simulink model "FG_Simulator"  (R2017b)
settings: Solver=ode45  StartTime=0  StopTime=20  FixedStep=0.0005  EnableMultiTasking=on
InitFcn:
  | isSim = 1;
  | 
  | PreFunctions.CustomInitFcn;
  | PreFunctions.simulationInitFcn
undefined symbols (not defined in the file): DiagnosticCodes, motorPositions, motorVelocities, pelvisPosition, pelvisVelocity, sample_time, X, Y, Z
libraries: sm_lib x170, nesl_utility x75, Contact_Forces_Lib x6, ComponentLibrary x5, Cassie_CommandBlock_Library_3 x1, Cassie_CommandBlock_Library_5 x1
(part 1 of 7)
settings Model: Creator=case  LastModifiedBy=81068
settings SolverCC: ZeroCrossControl=DisableAll  InsertRTBMode=Always
settings DataIOCC: SaveOutput=off  SignalLogging=off  DSMLogging=off  SaveTime=off
settings OptimizationCC: DefaultParameterBehavior=Inlined  UseFloatMulNetSlope=on  InlineInvariantSignals=on  EfficientFloat2IntCast=on  LifeSpan=inf  SimCompilerOptimization=on  AccelVerboseBuild=on
settings DebuggingCC: ReadBeforeWriteMsg=DisableAll  WriteAfterWriteMsg=DisableAll  WriteAfterReadMsg=DisableAll  ParameterUnderflowMsg=error  ParameterTunabilityLossMsg=error  UniqueDataStoreMsg=error  AllowSymbolicDim=off  StrictBusMsg=ErrorOnBusTreatedAsVector  SFUnexpectedBacktrackingDiag=warning  SFNoUnconditionalDefaultTransitionDiag=warning  SFExecutionAtInitializationDiag=none
settings HardwareCC: TargetBitPerPointer=64  TargetBitPerSizeT=64  TargetBitPerPtrDiffT=64  TargetLongLongMode=on  TargetIntDivRoundTo=Zero  TargetEndianess=LittleEndian  TargetWordSize=64  TargetHWDeviceType=MATLAB Host  ProdEqTarget=off
settings ModelReferenceCC: EnableParallelModelReferenceBuilds=on  ModelReferenceNumInstancesAllowed=Zero  ModelReferenceMinAlgLoopOccurrences=on  PropagateSignalLabelsOutOfModel=off
settings SFSimCC: SimUserIncludeDirs=$root_dir$\CustomCodes\utils\funcs\KinDyn200511_221619
settings SFSimCC: SimUserSources=|
  | R_LeftAbductionJoint_src.c
  | R_LeftThighJoint_src.c
  | R_RightAbductionJoint_src.c
  | R_RightThighJoint_src.c
  | 
  | AMworld_about_pA_src.c
  | 
  | Jb_BasePosX_src.c
  | Jb_BasePosY_src.c
  | Jb_BasePosZ_src.c
  | Jb_BaseRotX_src.c
  | Jb_BaseRotY_src.c
  | Jb_BaseRotZ_src.c
  | Jb_LeftAbductionJoint_src.c
  | Jb_LeftAnkleJoint_src.c
  | Jb_LeftHip_src.c
  | Jb_LeftKneeJoint_src.c
  | Jb_LeftKneeSpringJoint_src.c
  | Jb_LeftKnee_src.c
  | Jb_LeftPelvisRotation_src.c
  | Jb_LeftRotationJoint_src.c
  | Jb_LeftShin_src.c
  | Jb_LeftTarsus_src.c
  | Jb_LeftThighJoint_src.c
  | Jb_LeftThigh_src.c
  | Jb_LeftToeBottomBack_src.c
  | Jb_LeftToeBottomFront_src.c
  | Jb_LeftToeBottom_src.c
  | Jb_LeftToeJoint_src.c
  | Jb_LeftToe_src.c
  | Jb_Pelvis_src.c
  | Jb_RightAbductionJoint_src.c
  | Jb_RightAnkleJoint_src.c
  | Jb_RightHip_src.c
  | Jb_RightKneeJoint_src.c
  | Jb_RightKneeSpringJoint_src.c
  | Jb_RightKnee_src.c
  | Jb_RightPelvisRotation_src.c
  | Jb_RightRotationJoint_src.c
  | Jb_RightShin_src.c
  | Jb_RightTarsus_src.c
  | Jb_RightThighJoint_src.c
  | Jb_RightThigh_src.c
  | Jb_RightToeBottomBack_src.c
  | Jb_RightToeBottomFront_src.c
  | Jb_RightToeBottom_src.c
  | Jb_RightToeJoint_src.c
  | Jb_RightToe_src.c
  | 
  | Jdq_AMworld_about_pA_src.c
  | 
  | 
  | Jp_COM_src.c
  | Jp_LeftAbductionJoint_src.c
  | Jp_LeftAnkleJoint_src.c
  | Jp_LeftHip_src.c
  | Jp_LeftKneeJoint_src.c
  | Jp_LeftKneeSpringJoint_src.c
  | Jp_LeftKnee_src.c
  | Jp_LeftPelvisRotation_src.c
  | Jp_LeftRotationJoint_src.c
  | Jp_LeftShin_src.c
  | Jp_LeftTarsus_src.c
  | Jp_LeftThighJoint_src.c
  | Jp_LeftThigh_src.c
  | Jp_LeftToeBottomBack_src.c
  | Jp_LeftToeBottomFront_src.c
  | Jp_LeftToeBottom_src.c
  | Jp_LeftToeJoint_src.c
  | Jp_LeftToe_src.c
  | Jp_Pelvis_src.c
  | Jp_RightAbductionJoint_src.c
  | Jp_RightAnkleJoint_src.c
  | Jp_RightHip_src.c
  | Jp_RightKneeJoint_src.c
  | Jp_RightKneeSpringJoint_src.c
  | Jp_RightKnee_src.c
  | Jp_RightPelvisRotation_src.c
  | Jp_RightRotationJoint_src.c
  | Jp_RightShin_src.c
  | Jp_RightTarsus_src.c
  | Jp_RightThighJoint_src.c
  | Jp_RightThigh_src.c
  | Jp_RightToeBottomBack_src.c
  | Jp_RightToeBottomFront_src.c
  | Jp_RightToeBottom_src.c
  | Jp_RightToeJoint_src.c
  | Jp_RightToe_src.c
  | 
  | p_BasePosX_src.c
  | p_BasePosY_src.c
  | p_BasePosZ_src.c
  | p_BaseRotX_src.c
  | p_BaseRotY_src.c
  | p_BaseRotZ_src.c
  | p_COM_src.c
  | p_LeftAbductionJoint_src.c
  | p_LeftAnkleJoint_src.c
  | p_LeftHip_src.c
  | p_LeftKneeJoint_src.c
  | p_LeftKneeSpringJoint_src.c
  | p_LeftKnee_src.c
  | p_LeftPelvisRotation_src.c
  | p_LeftRotationJoint_src.c
  | p_LeftShin_src.c
  | p_LeftTarsus_src.c
  | p_LeftThighJoint_src.c
  | p_LeftThigh_src.c
  | p_LeftToeBottomBack_src.c
  | p_LeftToeBottomFront_src.c
  | p_LeftToeBottom_src.c
  | p_LeftToeJoint_src.c
  | p_LeftToe_src.c
  | p_Pelvis_src.c
  | p_RightAbductionJoint_src.c
  | p_RightAnkleJoint_src.c
  | p_RightHip_src.c
  | p_RightKneeJoint_src.c
  | p_RightKneeSpringJoint_src.c
  | p_RightKnee_src.c
  | p_RightPelvisRotation_src.c
  | p_RightRotationJoint_src.c
  | p_RightShin_src.c
  | p_RightTarsus_src.c
  | p_RightThighJoint_src.c
  | p_RightThigh_src.c
  | p_RightToeBottomBack_src.c
  | p_RightToeBottomFront_src.c
  | p_RightToeBottom_src.c
  | p_RightToeJoint_src.c
  | p_RightToe_src.c
  | 
  | T_LeftToeBottomBack_src.c
  | T_LeftToeBottomFront_src.c
  | T_LeftToeBottom_src.c
  | T_RightToeBottomBack_src.c
  | T_RightToeBottomFront_src.c
  | T_RightToeBottom_src.c
  | 
  | J_LL_Left_src.c
  | J_LL_Right_src.c
  | LL_Left_src.c
  | LL_Right_src.c
settings RTWCC: Description=Generic Real-Time Target  RTWUseSimCustomCode=on  CustomInclude=$root_dir$\CustomCodes\utils\funcs\KinDyn200511_221619  BuildConfiguration=Faster Runs  CheckMdlBeforeBuild=Warning
settings RTWCC: CustomSource=|
  | R_LeftAbductionJoint_src.c
  | R_LeftThighJoint_src.c
  | R_RightAbductionJoint_src.c
  | R_RightThighJoint_src.c
  | 
  | AMworld_about_pA_src.c
  | 
  | Jb_BasePosX_src.c
  | Jb_BasePosY_src.c
  | Jb_BasePosZ_src.c
  | Jb_BaseRotX_src.c
  | Jb_BaseRotY_src.c
  | Jb_BaseRotZ_src.c
  | Jb_LeftAbductionJoint_src.c
  | Jb_LeftAnkleJoint_src.c
  | Jb_LeftHip_src.c
  | Jb_LeftKneeJoint_src.c
  | Jb_LeftKneeSpringJoint_src.c
  | Jb_LeftKnee_src.c
  | Jb_LeftPelvisRotation_src.c
  | Jb_LeftRotationJoint_src.c
  | Jb_LeftShin_src.c
  | Jb_LeftTarsus_src.c
  | Jb_LeftThighJoint_src.c
  | Jb_LeftThigh_src.c
  | Jb_LeftToeBottomBack_src.c
  | Jb_LeftToeBottomFront_src.c
  | Jb_LeftToeBottom_src.c
  | Jb_LeftToeJoint_src.c
  | Jb_LeftToe_src.c
  | Jb_Pelvis_src.c
  | Jb_RightAbductionJoint_src.c
  | Jb_RightAnkleJoint_src.c
  | Jb_RightHip_src.c
  | Jb_RightKneeJoint_src.c
  | Jb_RightKneeSpringJoint_src.c
  | Jb_RightKnee_src.c
  | Jb_RightPelvisRotation_src.c
  | Jb_RightRotationJoint_src.c
  | Jb_RightShin_src.c
  | Jb_RightTarsus_src.c
  | Jb_RightThighJoint_src.c
  | Jb_RightThigh_src.c
  | Jb_RightToeBottomBack_src.c
  | Jb_RightToeBottomFront_src.c
  | Jb_RightToeBottom_src.c
  | Jb_RightToeJoint_src.c
  | Jb_RightToe_src.c
  | 
  | Jdq_AMworld_about_pA_src.c
  | 
  | 
  | Jp_COM_src.c
  | Jp_LeftAbductionJoint_src.c
  | Jp_LeftAnkleJoint_src.c
  | Jp_LeftHip_src.c
  | Jp_LeftKneeJoint_src.c
  | Jp_LeftKneeSpringJoint_src.c
  | Jp_LeftKnee_src.c
  | Jp_LeftPelvisRotation_src.c
  | Jp_LeftRotationJoint_src.c
  | Jp_LeftShin_src.c
  | Jp_LeftTarsus_src.c
  | Jp_LeftThighJoint_src.c
  | Jp_LeftThigh_src.c
  | Jp_LeftToeBottomBack_src.c
  | Jp_LeftToeBottomFront_src.c
  | Jp_LeftToeBottom_src.c
  | Jp_LeftToeJoint_src.c
  | Jp_LeftToe_src.c
  | Jp_Pelvis_src.c
  | Jp_RightAbductionJoint_src.c
  | Jp_RightAnkleJoint_src.c
  | Jp_RightHip_src.c
  | Jp_RightKneeJoint_src.c
  | Jp_RightKneeSpringJoint_src.c
  | Jp_RightKnee_src.c
  | Jp_RightPelvisRotation_src.c
  | Jp_RightRotationJoint_src.c
  | Jp_RightShin_src.c
  | Jp_RightTarsus_src.c
  | Jp_RightThighJoint_src.c
  | Jp_RightThigh_src.c
  | Jp_RightToeBottomBack_src.c
  | Jp_RightToeBottomFront_src.c
  | Jp_RightToeBottom_src.c
  | Jp_RightToeJoint_src.c
  | Jp_RightToe_src.c
  | 
  | p_BasePosX_src.c
  | p_BasePosY_src.c
  | p_BasePosZ_src.c
  | p_BaseRotX_src.c
  | p_BaseRotY_src.c
  | p_BaseRotZ_src.c
  | p_COM_src.c
  | p_LeftAbductionJoint_src.c
  | p_LeftAnkleJoint_src.c
  | p_LeftHip_src.c
  | p_LeftKneeJoint_src.c
  | p_LeftKneeSpringJoint_src.c
  | p_LeftKnee_src.c
  | p_LeftPelvisRotation_src.c
  | p_LeftRotationJoint_src.c
  | p_LeftShin_src.c
  | p_LeftTarsus_src.c
  | p_LeftThighJoint_src.c
  | p_LeftThigh_src.c
  | p_LeftToeBottomBack_src.c
  | p_LeftToeBottomFront_src.c
  | p_LeftToeBottom_src.c
  | p_LeftToeJoint_src.c
  | p_LeftToe_src.c
  | p_Pelvis_src.c
  | p_RightAbductionJoint_src.c
  | p_RightAnkleJoint_src.c
  | p_RightHip_src.c
  | p_RightKneeJoint_src.c
  | p_RightKneeSpringJoint_src.c
  | p_RightKnee_src.c
  | p_RightPelvisRotation_src.c
  | p_RightRotationJoint_src.c
  | p_RightShin_src.c
  | p_RightTarsus_src.c
  | p_RightThighJoint_src.c
  | p_RightThigh_src.c
  | p_RightToeBottomBack_src.c
  | p_RightToeBottomFront_src.c
  | p_RightToeBottom_src.c
  | p_RightToeJoint_src.c
  | p_RightToe_src.c
  | 
  | T_LeftToeBottomBack_src.c
  | T_LeftToeBottomFront_src.c
  | T_LeftToeBottom_src.c
  | T_RightToeBottomBack_src.c
  | T_RightToeBottomFront_src.c
  | T_RightToeBottom_src.c
  | 
  | J_LL_Left_src.c
  | J_LL_Right_src.c
  | LL_Left_src.c
  | LL_Right_src.c
settings CodeAppCC: GenerateComments=off  SimulinkBlockComments=off
settings GRTTargetCC: MatFileLogging=off  MultiInstanceERTCode=on  CodeInterfacePackaging=Reusable function  SupportNonFinite=off  GenerateAllocFcn=on
settings ConfigComp: CovMetricSettings=dw  CovHtmlReporting=on  CovSaveCumulativeToWorkspaceVar=on  CovSaveSingleToWorkspaceVar=on  CovExternalEMLEnable=off
settings SimscapeCC: SimscapeNormalizeSystem=off
settings DiagnosticsConfigSet: SimMechanicsRigidlyBoundBlock=warning
settings ExplorerConfigSet: InternalSimMechanicsExplorerSettings="<ExplorerConfiguration><canonicalview>default</canonicalview><AnimationSetting><BasePlaybackSpeed>1.0</BasePlaybackSpeed><PlaybackSpeedFactor>1.0</PlaybackSpeedFactor></AnimationSetting><TilePanel><TileInfo><Tiles Columns=\"1\" Count=\"1\" Rows=\"1\"><Column Weight=\"1\"/><Row Weight=\"1\"/><Tile Height=\"1\" Width=\"1\" X=\"0\" Y=\"0\"/></Tiles></TileInfo><SceneInfo><SceneViewer><BGColor><R>0.60000002384185791</R><G>0.60000002384185791</G><B>0.60000002384185791</B></BGColor><Camera><DoPerspective>off</DoPerspective><Position><X>-35.4589435173178984</X><Y>-0.0500115168093022214</Y><Z>0.273628552513051182</Z></Position><Center><X>1.71805707793737383e-06</X><Y>-0.0500115168093022214</Y><Z>0.273628552513051182</Z></Center><Up><X>0</X><Y>0</Y><Z>1</Z></Up><ViewLimDist>1</ViewLimDist><YLim>8.2670531882207996</YLim><XLim>14.7535103051325045</XLim></Camera></SceneViewer></SceneInfo></TilePanel><MechEditorPanel><Cameras><Camera><Id>Camera1</Id><Value><Name>Tracking Camera</Name><NativeCamera><PositionTrackingFeature>Cassie.Cassie_Simulation.World.Tracking_Camera.F</PositionTrackingFeature><CenterTrackingFeature>Cassie.Cassie_Simulation.World.Tracking_Camera_Target.F</CenterTrackingFeature><UpVectorTrackingFeature>Cassie.Cassie_Simulation.World.Tracking_Camera_Target.F</UpVectorTrackingFeature><CenterTrackingOrigin>on</CenterTrackingOrigin><UpVectorTrackingDirection>+Z</UpVectorTrackingDirection></NativeCamera></Value></Camera><Camera><Id>Camera2</Id><Value><Name>Fixed Camera</Name><NativeCamera><PositionTrackingFeature>Cassie.Cassie_Simulation.World.Fixed_Camera.F</PositionTrackingFeature><CenterTrackingFeature>Cassie.Cassie_Simulation.World.Fixed_Camera_Target.F</CenterTrackingFeature><UpVectorTrackingFeature>Cassie.Cassie_Simulation.World.Fixed_Camera_Target.F</UpVectorTrackingFeature><CenterTrackingOrigin>on</CenterTrackingOrigin><UpVectorTrackingDirection>+Z</UpVectorTrackingDirection></NativeCamera></Value></Camera><Camera><Id>Camera3</Id><Value><Name>tracking camera positive y</Name><NativeCamera><PositionTrackingFeature>Cassie.Cassie_Simulation.Cassie_Pelvis_World</PositionTrackingFeature><CenterTrackingFeature/><UpVectorTrackingFeature/><CenterTrackingOrigin>off</CenterTrackingOrigin><CenterTrackingDirection>+Y</CenterTrackingDirection><UpVectorTrackingDirection>+Z</UpVectorTrackingDirection></NativeCamera></Value></Camera></Cameras><GfxPanelCameraMap/><VideoCreator><PlaybackSpeedRatio>1.0</PlaybackSpeedRatio><FrameRate>30</FrameRate><VideoFormat>MPEG-4</VideoFormat><FrameSize>[1920 1080]</FrameSize></VideoCreator></MechEditorPanel></ExplorerConfiguration>"

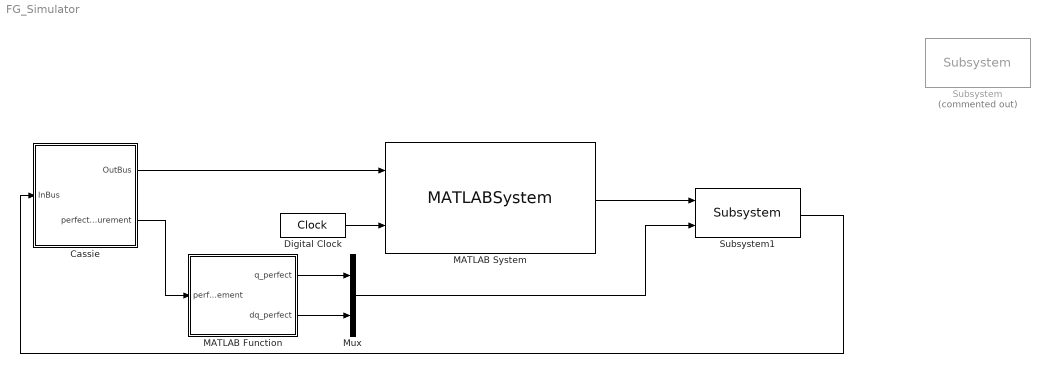
== system FG_Simulator ==
  Cassie : Subsystem  AncestorBlock=CassieLibrary/Simulation/Cassie  InitFcn=|  StartFcn=|  StopFcn=|
      InitFcn=|
      | % Start clock at initialization (used for computing real time performance)
      | initTime = tic;
      | 
      | % Import bus definitions
      | CassieModule.importBuses;
      StartFcn=|
      | % Store build time
      | buildTime = toc(initTime);
      StopFcn=|
      | % Store computation time
      | computationTime = toc(initTime) - buildTime;
      | 
      | % Get simulation time
      | simulationTime = get_param(bdroot, 'SimulationTime');
      | 
      | % Compute real time performance
      | percentRealTime = 100*simulationTime/computationTime;
      | 
      | % Display
      | fprintf('Build time: %0.2f seconds \n', buildTime);
      | fprintf('Simulation time: %0.2f seconds \n', simulationTime);
      | fprintf('Computation time: %0.2f seconds \n', computationTime);
      | fprintf('Performance: %0.2f%% real time \n', percentRealTime);
      mask Display: image('Cassie.png');
  Digital Clock : DigitalClock  SampleTime=sample_time
  MATLAB Function : MATLAB Function  TreatAsAtomicUnit=on
  MATLAB System : MATLABSystem  System=RemoteSpoofer  SimulateUsing=Interpreted execution
      mask Type: RemoteSpoofer
      mask Display:
      | disp('RemoteSpoofer');
      | port_label('input',1,'cassieOutputs');
      | port_label('input',2,'t');
      | port_label('output',1,'cassieOutputs');
  Mux : Mux  Inputs=2
  Subsystem : Cassie_CommandBlock_Library_3/Subsystem  Commented=on
  Subsystem1 : Cassie_CommandBlock_Library_5/Subsystem
  wires:
  Cassie/1(OutBus) -> MATLAB System/1
  Digital Clock/1 -> MATLAB System/2
  MATLAB System/1 -> Subsystem1/1
  Subsystem1/1 -> Cassie/1(InBus)
  Cassie/2(perfect measurement) -> MATLAB Function/1(perfect_measurement)
  MATLAB Function/1(q_perfect) -> Mux/1
  MATLAB Function/2(dq_perfect) -> Mux/2
  Mux/1 -> Subsystem1/2

== system FG_Simulator/Cassie ==
  InBus : Inport  OutDataTypeStr=Bus: CassieUserInBus
  Cassie Core MATLAB System : MATLABSystem  System=CassieCoreSim  SimulateUsing=Code generation
      mask Type: CassieCoreSim
      mask Display: disp('CassieCoreSim');
  Cassie Simulation : Subsystem  AncestorBlock=CassieLibrary/Simulation/Cassie Simulation
      mask Display: image('Cassie.png');
  Delay : Delay  DelayLength=1
  Rate Transition : RateTransition  OutPortSampleTime=0.0005
  Signal Conversion : SignalConversion  ConversionOutput=Nonvirtual bus  OutDataTypeStr=Bus: CassieOutBus  OverrideOpt=off
  OutBus : Outport  OutDataTypeStr=Bus: CassieOutBus
  perfect measurement : Outport  Port=2
  wires:
  Signal Conversion/1 -> Cassie Core MATLAB System/2, OutBus/1
  Cassie Simulation/1(OutBus) -> Rate Transition/1
  Rate Transition/1 -> Signal Conversion/1
  Delay/1 -> Cassie Simulation/1(InBus)
  Cassie Core MATLAB System/1 -> Delay/1
  InBus/1 -> Cassie Core MATLAB System/1
  Cassie Simulation/2(perfect measurement) -> perfect measurement/1

== system FG_Simulator/Cassie/Cassie Simulation ==
  Bus Element In2 : Inport  PortName=InBus  Element=leftLeg
  Bus Element In3 : Inport  PortName=InBus  Element=rightLeg
  Bus Element In1 : Inport  PortName=InBus  Element=pelvis
  Cassie Left Leg : Subsystem  AncestorBlock=CassieLibrary/Simulation/Cassie Leg  mask{config=Left, motorPositions=motorPositions(1:5), motorVelocities=motorVelocities(1:5)}
      mask prompts: config "Configuration:"; motorPositions "Initial Motor Positions (rad):"; motorVelocities "Initial Motor Velocities (rad/s):"
      mask init:
      | d = CassieDescriptor;
      | bodyIndex = @(s, name) find(arrayfun(@(s) isequal(s.name, name), s));
      | 
      | switch config
      |   case 1 % Left
      |     % Hip Roll
      |     b = d(bodyIndex(d, 'left-hip-roll'));
      |     set_param([gcb, '/Hip Roll Solid'], 'ExtGeomFileName', [b.name '.stl']);
      |     set_param([gcb, '/Hip Roll Solid'], 'Mass', mat2str(b.m));
      |     set_param([gcb, '/Hip Roll Solid'], 'CenterOfMass', mat2str(b.c));
      |     set_param([gcb, '/Hip Roll Solid'], 'MomentsOfInertia', mat2str(b.Ic(1:3)));
      |     set_param([gcb, '/Hip Roll Solid'], 'ProductsOfInertia', mat2str(b.Ic(4:6)));
      |     %set_param([gcb, '/Pelvis to Hip Roll'], 'TranslationCartesianOffset', mat2str(b.r));
      |     %set_param([gcb, '/Pelvis to Hip Roll'], 'RotationMatrix', mat2str(b.R));
      |     
      |     % Hip Yaw
      |     b = d(bodyIndex(d, 'left-hip-yaw'));
      |     set_param([gcb, '/Hip Yaw Solid'], 'ExtGeomFileName', [b.name '.stl']);
      |     set_param([gcb, '/Hip Yaw Solid'], 'Mass', mat2str(b.m));
      |     set_param([gcb, '/Hip Yaw Solid'], 'CenterOfMass', mat2str(b.c));
      |     set_param([gcb, '/Hip Yaw Solid'], 'MomentsOfInertia', mat2str(b.Ic(1:3)));
      |     set_param([gcb, '/Hip Yaw Solid'], 'ProductsOfInertia', mat2str(b.Ic(4:6)));
      |     set_param([gcb, '/Hip Roll to Hip Yaw'], 'TranslationCartesianOffset', mat2str(b.r));
      |     set_param([gcb, '/Hip Roll to Hip Yaw'], 'RotationMatrix', mat2str(b.R));
      |     
      |     % Hip Pitch
      |     b = d(bodyIndex(d, 'left-hip-pitch'));
      |     set_param([gcb, '/Hip Pitch Solid'], 'ExtGeomFileName', [b.name '.stl']);
      |     set_param([gcb, '/Hip Pitch Solid'], 'Mass', mat2str(b.m));
      |     set_param([gcb, '/Hip Pitch Solid'], 'CenterOfMass', mat2str(b.c));
      |     set_param([gcb, '/Hip Pitch Solid'], 'MomentsOfInertia', mat2str(b.Ic(1:3)));
      |     set_param([gcb, '/Hip Pitch Solid'], 'ProductsOfInertia', mat2str(b.Ic(4:6)));
      |     set_param([gcb, '/Hip Yaw to Hip Pitch'], 'TranslationCartesianOffset', mat2str(b.r));
      |     set_param([gcb, '/Hip Yaw to Hip Pitch'], 'RotationMatrix', mat2str(b.R));
      |     
      |     % Achilles Rod
      |     b = d(bodyIndex(d, 'left-achilles-rod'));
      |     set_param([gcb, '/Achilles Rod Solid'], 'ExtGeomFileName', [b.name '.stl']);
      |     set_param([gcb, '/Achilles Rod Solid'], 'Mass', mat2str(b.m));
      |     set_param([gcb, '/Achilles Rod Solid'], 'CenterOfMass', mat2str(b.c));
      |     set_param([gcb, '/Achilles Rod Solid'], 'MomentsOfInertia', mat2str(b.Ic(1:3)));
      |     set_param([gcb, '/Achilles Rod Solid'], 'ProductsOfInertia', mat2str(b.Ic(4:6)));
      |     set_param([gcb, '/Hip Pitch to Achilles Rod'], 'TranslationCartesianOffset', mat2str(b.r));
      |     set_param([gcb, '/Hip Pitch to Achilles Rod'], 'RotationMatrix', mat2str(b.R));
      |     
      |     % Knee
      |     b = d(bodyIndex(d, 'left-knee'));
      |     set_param([gcb, '/Knee Solid'], 'ExtGeomFileName', [b.name '.stl']);
      |     set_param([gcb, '/Knee Solid'], 'Mass', mat2str(b.m));
      |     set_param([gcb, '/Knee Solid'], 'CenterOfMass', mat2str(b.c));
      |     set_param([gcb, '/Knee Solid'], 'MomentsOfInertia', mat2str(b.Ic(1:3)));
      |     set_param([gcb, '/Knee Solid'], 'ProductsOfInertia', mat2str(b.Ic(4:6)));
      |     set_param([gcb, '/Hip Pitch to Knee'], 'TranslationCartesianOffset', mat2str(b.r));
      |     set_param([gcb, '/Hip Pitch to Knee'], 'RotationMatrix', mat2str(b.R));
      |     
      |     % Knee Spring
      |     b = d(bodyIndex(d, 'left-knee-spring'));
      |     set_param([gcb, '/Knee Spring Solid'], 'ExtGeomFileName', [b.name '.stl']);
      |     set_param([gcb, '/Knee Spring Solid'], 'Mass', mat2str(b.m));
      |     set_param([gcb, '/Knee Spring Solid'], 'CenterOfMass', mat2str(b.c));
      |     set_param([gcb, '/Knee Spring Solid'], 'MomentsOfInertia', mat2str(b.Ic(1:3)));
      |     set_param([gcb, '/Knee Spring Solid'], 'ProductsOfInertia', mat2str(b.Ic(4:6)));
      |     set_param([gcb, '/Knee to Knee Spring'], 'TranslationCartesianOffset', mat2str(b.r));
      |     set_param([gcb, '/Knee to Knee Spring'], 'RotationMatrix', mat2str(b.R));
      |     
      |     % Shin
      |     b = d(bodyIndex(d, 'left-shin'));
      |     set_param([gcb, '/Shin Solid'], 'ExtGeomFileName', [b.name '.stl']);
      |     set_param([gcb, '/Shin Solid'], 'Mass', mat2str(b.m));
      |     set_param([gcb, '/Shin Solid'], 'CenterOfMass', mat2str(b.c));
      |     set_param([gcb, '/Shin Solid'], 'MomentsOfInertia', mat2str(b.Ic(1:3)));
      |     set_param([gcb, '/Shin Solid'], 'ProductsOfInertia', mat2str(b.Ic(4:6)));
      |     set_param([gcb, '/Knee to Shin'], 'TranslationCartesianOffset', mat2str(b.r));
      |     set_param([gcb, '/Knee to Shin'], 'RotationMatrix', mat2str(b.R));
      |     
      |     % Tarsus
      |     b = d(bodyIndex(d, 'left-tarsus'));
      |     set_param([gcb, '/Tarsus Solid'], 'ExtGeomFileName', [b.name '.stl']);
      |     set_param([gcb, '/Tarsus Solid'], 'Mass', mat2str(b.m));
      |     set_param([gcb, '/Tarsus Solid'], 'CenterOfMass', mat2str(b.c));
      |     set_param([gcb, '/Tarsus Solid'], 'MomentsOfInertia', mat2str(b.Ic(1:3)));
      |     set_param([gcb, '/Tarsus Solid'], 'ProductsOfInertia', mat2str(b.Ic(4:6)));
      |     set_param([gcb, '/Shin to Tarsus'], 'TranslationCartesianOffset', mat2str(b.r));
      |     set_param([gcb, '/Shin to Tarsus'], 'RotationMatrix', mat2str(b.R));
      |     
      |     % Heel Spring
      |     b = d(bodyIndex(d, 'left-heel-spring'));
      |     set_param([gcb, '/Heel Spring Solid'], 'ExtGeomFileName', [b.name '.stl']);
      |     set_param([gcb, '/Heel Spring Solid'], 'Mass', mat2str(b.m));
      |     set_param([gcb, '/Heel Spring Solid'], 'CenterOfMass', mat2str(b.c));
      |     set_param([gcb, '/Heel Spring Solid'], 'MomentsOfInertia', mat2str(b.Ic(1:3)));
      |     set_param([gcb, '/Heel Spring Solid'], 'ProductsOfInertia', mat2str(b.Ic(4:6)));
      |     set_param([gcb, '/Tarsus to Heel Spring'], 'TranslationCartesianOffset', mat2str(b.r));
      |     set_param([gcb, '/Tarsus to Heel Spring'], 'RotationMatrix', mat2str(b.R));
      |     
      |     % Foot Crank
      |     b = d(bodyIndex(d, 'left-foot-crank'));
      |     set_param([gcb, '/Foot Crank Solid'], 'ExtGeomFileName', [b.name '.stl']);
      |     set_param([gcb, '/Foot Crank Solid'], 'Mass', mat2str(b.m));
      |     set_param([gcb, '/Foot Crank Solid'], 'CenterOfMass', mat2str(b.c));
      |     set_param([gcb, '/Foot Crank Solid'], 'MomentsOfInertia', mat2str(b.Ic(1:3)));
      |     set_param([gcb, '/Foot Crank Solid'], 'ProductsOfInertia', mat2str(b.Ic(4:6)));
      |     set_param([gcb, '/Tarsus to Foot Crank'], 'TranslationCartesianOffset', mat2str(b.r));
      |     set_param([gcb, '/Tarsus to Foot Crank'], 'RotationMatrix', mat2str(b.R));
      |     
      |     % Plantar Rod
      |     b = d(bodyIndex(d, 'left-plantar-rod'));
      |     set_param([gcb, '/Plantar Rod Solid'], 'ExtGeomFileName', [b.name '.stl']);
      |     set_param([gcb, '/Plantar Rod Solid'], 'Mass', mat2str(b.m));
      |     set_param([gcb, '/Plantar Rod Solid'], 'CenterOfMass', mat2str(b.c));
      |     set_param([gcb, '/Plantar Rod Solid'], 'MomentsOfInertia', mat2str(b.Ic(1:3)));
      |     set_param([gcb, '/Plantar Rod Solid'], 'ProductsOfInertia', mat2str(b.Ic(4:6)));
      |     set_param([gcb, '/Foot Crank to Plantar Rod'], 'TranslationCartesianOffset', mat2str(b.r));
      |     set_param([gcb, '/Foot Crank to Plantar Rod'], 'RotationMatrix', mat2str(b.R));
      |     
      |     % Foot
      |     b = d(bodyIndex(d, 'left-foot'));
      |     set_param([gcb, '/Foot Solid'], 'ExtGeomFileName', [b.name '.stl']);
      |     set_param([gcb, '/Foot Solid'], 'Mass', mat2str(b.m));
      |     set_param([gcb, '/Foot Solid'], 'CenterOfMass', mat2str(b.c));
      |     set_param([gcb, '/Foot Solid'], 'MomentsOfInertia', mat2str(b.Ic(1:3)));
      |     set_param([gcb, '/Foot Solid'], 'ProductsOfInertia', mat2str(b.Ic(4:6)));
      |     set_param([gcb, '/Tarsus to Foot'], 'TranslationCartesianOffset', mat2str(b.r));
      |     set_param([gcb, '/Tarsus to Foot'], 'RotationMatrix', mat2str(b.R));
      |     
      |     % Foot Pin
      |     %b = d(bodyIndex(d, 'left-foot-pin'));
      |     set_param([gcb, '/Foot to Foot Pin'], 'TranslationCartesianOffset', mat2str([0.055 0 0.00776]));
      |     set_param([gcb, '/Foot to Foot Pin'], 'RotationMatrix', mat2str(eye(3)));
      |     
      |     % Midfoot
      |     %b = d(bodyIndex(d, 'left-mid-foot'));
      |     set_param([gcb, '/Foot to Midfoot'], 'TranslationCartesianOffset', mat2str([0.01762 0.05219 0]));
      |     set_param([gcb, '/Foot to Midfoot'], 'RotationMatrix', mat2str([-0.766044443118978 0 -0.642787609686539;0.642787609686539 0 -0.766044443118978;0 -1 0]));
      |     
      |   case 2 % Right
      |     % Hip Roll
      |     b = d(bodyIndex(d, 'right-hip-roll'));
      |     set_param([gcb, '/Hip Roll Solid'], 'ExtGeomFileName', [b.name '.stl']);
      |     set_param([gcb, '/Hip Roll Solid'], 'Mass', mat2str(b.m));
      |     set_param([gcb, '/Hip Roll Solid'], 'CenterOfMass', mat2str(b.c));
      |     set_param([gcb, '/Hip Roll Solid'], 'MomentsOfInertia', mat2str(b.Ic(1:3)));
      |     set_param([gcb, '/Hip Roll Solid'], 'ProductsOfInertia', mat2str(b.Ic(4:6)));
      |     %set_param([gcb, '/Pelvis to Hip Roll'], 'TranslationCartesianOffset', mat2str(b.r));
      |     %set_param([gcb, '/Pelvis to Hip Roll'], 'RotationMatrix', mat2str(b.R));
      |     
      |     % Hip Yaw
      |     b = d(bodyIndex(d, 'right-hip-yaw'));
      |     set_param([gcb, '/Hip Yaw Solid'], 'ExtGeomFileName', [b.name '.stl']);
      |     set_param([gcb, '/Hip Yaw Solid'], 'Mass', mat2str(b.m));
      |     set_param([gcb, '/Hip Yaw Solid'], 'CenterOfMass', mat2str(b.c));
      |     set_param([gcb, '/Hip Yaw Solid'], 'MomentsOfInertia', mat2str(b.Ic(1:3)));
      |     set_param([gcb, '/Hip Yaw Solid'], 'ProductsOfInertia', mat2str(b.Ic(4:6)));
      |     set_param([gcb, '/Hip Roll to Hip Yaw'], 'TranslationCartesianOffset', mat2str(b.r));
      |     set_param([gcb, '/Hip Roll to Hip Yaw'], 'RotationMatrix', mat2str(b.R));
      |     
      |     % Hip Pitch
      |     b = d(bodyIndex(d, 'right-hip-pitch'));
      |     set_param([gcb, '/Hip Pitch Solid'], 'ExtGeomFileName', [b.name '.stl']);
      |     set_param([gcb, '/Hip Pitch Solid'], 'Mass', mat2str(b.m));
      |     set_param([gcb, '/Hip Pitch Solid'], 'CenterOfMass', mat2str(b.c));
      |     set_param([gcb, '/Hip Pitch Solid'], 'MomentsOfInertia', mat2str(b.Ic(1:3)));
      |     set_param([gcb, '/Hip Pitch Solid'], 'ProductsOfInertia', mat2str(b.Ic(4:6)));
      |     set_param([gcb, '/Hip Yaw to Hip Pitch'], 'TranslationCartesianOffset', mat2str(b.r));
      |     set_param([gcb, '/Hip Yaw to Hip Pitch'], 'RotationMatrix', mat2str(b.R));
      |     
      |     % Achilles Rod
      |     b = d(bodyIndex(d, 'right-achilles-rod'));
      |     set_param([gcb, '/Achilles Rod Solid'], 'ExtGeomFileName', [b.name '.stl']);
      |     set_param([gcb, '/Achilles Rod Solid'], 'Mass', mat2str(b.m));
      |     set_param([gcb, '/Achilles Rod Solid'], 'CenterOfMass', mat2str(b.c));
      |     set_param([gcb, '/Achilles Rod Solid'], 'MomentsOfInertia', mat2str(b.Ic(1:3)));
      |     set_param([gcb, '/Achilles Rod Solid'], 'ProductsOfInertia', mat2str(b.Ic(4:6)));
      |     set_param([gcb, '/Hip Pitch to Achilles Rod'], 'TranslationCartesianOffset', mat2str(b.r));
      |     set_param([gcb, '/Hip Pitch to Achilles Rod'], 'RotationMatrix', mat2str(b.R));
      |     
      |     % Knee
      |     b = d(bodyIndex(d, 'right-knee'));
      |     set_param([gcb, '/Knee Solid'], 'ExtGeomFileName', [b.name '.stl']);
      |     set_param([gcb, '/Knee Solid'], 'Mass', mat2str(b.m));
      |     set_param([gcb, '/Knee Solid'], 'CenterOfMass', mat2str(b.c));
      |     set_param([gcb, '/Knee Solid'], 'MomentsOfInertia', mat2str(b.Ic(1:3)));
      |     set_param([gcb, '/Knee Solid'], 'ProductsOfInertia', mat2str(b.Ic(4:6)));
      |     set_param([gcb, '/Hip Pitch to Knee'], 'TranslationCartesianOffset', mat2str(b.r));
      |     set_param([gcb, '/Hip Pitch to Knee'], 'RotationMatrix', mat2str(b.R));
      |     
      |     % Knee Spring
      |     b = d(bodyIndex(d, 'right-knee-spring'));
      |     set_param([gcb, '/Knee Spring Solid'], 'ExtGeomFileName', [b.name '.stl']);
      |     set_param([gcb, '/Knee Spring Solid'], 'Mass', mat2str(b.m));
      |     set_param([gcb, '/Knee Spring Solid'], 'CenterOfMass', mat2str(b.c));
      |     set_param([gcb, '/Knee Spring Solid'], 'MomentsOfInertia', mat2str(b.Ic(1:3)));
      |     set_param([gcb, '/Knee Spring Solid'], 'ProductsOfInertia', mat2str(b.Ic(4:6)));
      |     set_param([gcb, '/Knee to Knee Spring'], 'TranslationCartesianOffset', mat2str(b.r));
      |     set_param([gcb, '/Knee to Knee Spring'], 'RotationMatrix', mat2str(b.R));
      |     
      |     % Shin
      |     b = d(bodyIndex(d, 'right-shin'));
      |     set_param([gcb, '/Shin Solid'], 'ExtGeomFileName', [b.name '.stl']);
      |     set_param([gcb, '/Shin Solid'], 'Mass', mat2str(b.m));
      |     set_param([gcb, '/Shin Solid'], 'CenterOfMass', mat2str(b.c));
      |     set_param([gcb, '/Shin Solid'], 'MomentsOfInertia', mat2str(b.Ic(1:3)));
      |     set_param([gcb, '/Shin Solid'], 'ProductsOfInertia', mat2str(b.Ic(4:6)));
      |     set_param([gcb, '/Knee to Shin'], 'TranslationCartesianOffset', mat2str(b.r));
      |     set_param([gcb, '/Knee to Shin'], 'RotationMatrix', mat2str(b.R));
      |     
      |     % Tarsus
      |     b = d(bodyIndex(d, 'right-tarsus'));
      |     set_param([gcb, '/Tarsus Solid'], 'ExtGeomFileName', [b.name '.stl']);
      |     set_param([gcb, '/Tarsus Solid'], 'Mass', mat2str(b.m));
      |     set_param([gcb, '/Tarsus Solid'], 'CenterOfMass', mat2str(b.c));
      |     set_param([gcb, '/Tarsus Solid'], 'MomentsOfInertia', mat2str(b.Ic(1:3)));
      |     set_param([gcb, '/Tarsus Solid'], 'ProductsOfInertia', mat2str(b.Ic(4:6)));
      |     set_param([gcb, '/Shin to Tarsus'], 'TranslationCartesianOffset', mat2str(b.r));
      |     set_param([gcb, '/Shin to Tarsus'], 'RotationMatrix', mat2str(b.R));
      |     
      |     % Heel Spring
      |     b = d(bodyIndex(d, 'right-heel-spring'));
      |     set_param([gcb, '/Heel Spring Solid'], 'ExtGeomFileName', [b.name '.stl']);
      |     set_param([gcb, '/Heel Spring Solid'], 'Mass', mat2str(b.m));
      |     set_param([gcb, '/Heel Spring Solid'], 'CenterOfMass', mat2str(b.c));
      |     set_param([gcb, '/Heel Spring Solid'], 'MomentsOfInertia', mat2str(b.Ic(1:3)));
      |     set_param([gcb, '/Heel Spring Solid'], 'ProductsOfInertia', mat2str(b.Ic(4:6)));
      |     set_param([gcb, '/Tarsus to Heel Spring'], 'TranslationCartesianOffset', mat2str(b.r));
      |     set_param([gcb, '/Tarsus to Heel Spring'], 'RotationMatrix', mat2str(b.R));
      |     
      |     % Foot Crank
      |     b = d(bodyIndex(d, 'right-foot-crank'));
      |     set_param([gcb, '/Foot Crank Solid'], 'ExtGeomFileName', [b.name '.stl']);
      |     set_param([gcb, '/Foot Crank Solid'], 'Mass', mat2str(b.m));
      |     set_param([gcb, '/Foot Crank Solid'], 'CenterOfMass', mat2str(b.c));
      |     set_param([gcb, '/Foot Crank Solid'], 'MomentsOfInertia', mat2str(b.Ic(1:3)));
      |     set_param([gcb, '/Foot Crank Solid'], 'ProductsOfInertia', mat2str(b.Ic(4:6)));
      |     set_param([gcb, '/Tarsus to Foot Crank'], 'TranslationCartesianOffset', mat2str(b.r));
      |     set_param([gcb, '/Tarsus to Foot Crank'], 'RotationMatrix', mat2str(b.R));
      |     
      |     % Plantar Rod
      |     b = d(bodyIndex(d, 'right-plantar-rod'));
      |     set_param([gcb, '/Plantar Rod Solid'], 'ExtGeomFileName', [b.name '.stl']);
      |     set_param([gcb, '/Plantar Rod Solid'], 'Mass', mat2str(b.m));
      |     set_param([gcb, '/Plantar Rod Solid'], 'CenterOfMass', mat2str(b.c));
      |     set_param([gcb, '/Plantar Rod Solid'], 'MomentsOfInertia', mat2str(b.Ic(1:3)));
      |     set_param([gcb, '/Plantar Rod Solid'], 'ProductsOfInertia', mat2str(b.Ic(4:6)));
      |     set_param([gcb, '/Foot Crank to Plantar Rod'], 'TranslationCartesianOffset', mat2str(b.r));
      |     set_param([gcb, '/Foot Crank to Plantar Rod'], 'RotationMatrix', mat2str(b.R));
      |     
      |     % Foot
      |     b = d(bodyIndex(d, 'right-foot'));
      |     set_param([gcb, '/Foot Solid'], 'ExtGeomFileName', [b.name '.stl']);
      |     set_param([gcb, '/Foot Solid'], 'Mass', mat2str(b.m));
      |     set_param([gcb, '/Foot Solid'], 'CenterOfMass', mat2str(b.c));
      |     set_param([gcb, '/Foot Solid'], 'MomentsOfInertia', mat2str(b.Ic(1:3)));
      |     set_param([gcb, '/Foot Solid'], 'ProductsOfInertia', mat2str(b.Ic(4:6)));
      |     set_param([gcb, '/Tarsus to Foot'], 'TranslationCartesianOffset', mat2str(b.r));
      |     set_param([gcb, '/Tarsus to Foot'], 'RotationMatrix', mat2str(b.R));
      |     
      |     % Foot Pin
      |     %b = d(bodyIndex(d, 'right-foot-pin'));
      |     set_param([gcb, '/Foot to Foot Pin'], 'TranslationCartesianOffset', mat2str([0.055 0 -0.00776]));
      |     set_param([gcb, '/Foot to Foot Pin'], 'RotationMatrix', mat2str(eye(3)));
      |     
      |     % Midfoot
      |     %b = d(bodyIndex(d, 'right-mid-foot'));
      |     set_param([gcb, '/Foot to Midfoot'], 'TranslationCartesianOffset', mat2str([0.01762 0.05219 0]));
      |     set_param([gcb, '/Foot to Midfoot'], 'RotationMatrix', mat2str([-0.766044443118978 0 -0.642787609686539;0.642787609686539 0 -0.766044443118978;0 -1 0]));
      | end % switch
      | 
      | % Check if block is not in library model
      | if ~bdIsLibrary(bdroot)
      |   % Construct discrete filter for velocity estimation
      |   dt = str2num(get_param(bdroot, 'FixedStep'));
      |   filter1 = ButterworthFilter(2);
      |   filter1.setTimeConstant(0.003, dt);
      |   filter2 = BackwardDifferencingFilter(2);
      |   filter2.setSampleTime(dt);
      |   filter3 = Filter(filter1, filter2, 'cascade');
      |   [a, b] = filter3.getCoefficients;
      |   
      |   % Set discrete filter coefficients    
      |   set_param([gcb '/Shin Filter'], 'a', mat2str(a));
      |   set_param([gcb '/Shin Filter'], 'b', mat2str(b));
      |   set_param([gcb '/Tarsus Filter'], 'a', mat2str(a));
      |   set_param([gcb '/Tarsus Filter'], 'b', mat2str(b));
      |   set_param([gcb '/Foot Filter'], 'a', mat2str(a));
      |   set_param([gcb '/Foot Filter'], 'b', mat2str(b));
      | end % if
      mask TypeOptions config: Left | Right
  Cassie Pelvis : Subsystem  AncestorBlock=CassieLibrary/Simulation/Cassie Pelvis
  Cassie Right Leg : Subsystem  AncestorBlock=CassieLibrary/Simulation/Cassie Leg  mask{config=Right, motorPositions=motorPositions(6:10), motorVelocities=motorVelocities(6:10)}
      mask prompts: config "Configuration:"; motorPositions "Initial Motor Positions (rad):"; motorVelocities "Initial Motor Velocities (rad/s):"
      mask init: same as FG_Simulator/Cassie/Cassie Simulation/Cassie Left Leg
      mask TypeOptions config: Left | Right
  Constant : Constant  Value=true
  Constant1 : Constant  Value=DiagnosticCodes(zeros(4,1))
  Manual Switch : ManualSwitch
  Manual Switch1 : ManualSwitch
  Mux : Mux  Inputs=9
  World : Subsystem  AncestorBlock=ComponentLibrary/Simulation/World
  Bus Element Out4 : Outport  PortName=OutBus  Element=pelvis
  Bus Element Out2 : Outport  PortName=OutBus  Element=leftLeg
  Bus Element Out3 : Outport  PortName=OutBus  Element=rightLeg
  Bus Element Out1 : Outport  PortName=OutBus  Element=isCalibrated
  Bus Element Out5 : Outport  PortName=OutBus  Element=messages
  perfect measurement : Outport  Port=2
  wires:
  Constant1/1 -> Bus Element Out5/1
  Constant/1 -> Bus Element Out1/1
  Bus Element In1/1 -> Cassie Pelvis/1(InBus)
  Cassie Right Leg/1(OutBus) -> Bus Element Out3/1
  Bus Element In2/1 -> Cassie Left Leg/1(InBus)
  Cassie Left Leg/1(OutBus) -> Bus Element Out2/1
  Bus Element In3/1 -> Cassie Right Leg/1(InBus)
  Cassie Pelvis/1(OutBus) -> Bus Element Out4/1
  Cassie Pelvis/2(LinearAccelerator) -> Mux/1
  Cassie Pelvis/3(Quaternion) -> Mux/2
  Cassie Pelvis/4(AngularVelocity) -> Mux/3
  Cassie Left Leg/2(pos) -> Mux/5
  Cassie Right Leg/2(pos) -> Mux/6
  Cassie Left Leg/3(vel) -> Mux/8
  Cassie Right Leg/3(vel) -> Mux/9
  Mux/1 -> perfect measurement/1
  World/1(base_pos) -> Manual Switch/2
  World/2(base_vel) -> Manual Switch1/2
  Cassie Pelvis/6(IMU_vel) -> Manual Switch1/1
  Cassie Pelvis/5(IMU_pos) -> Manual Switch/1
  Manual Switch/1 -> Mux/4
  Manual Switch1/1 -> Mux/7
  connections:
  World/RConn1 -- Cassie Pelvis/LConn1
  Cassie Left Leg/LConn1 -- Cassie Pelvis/RConn1
  Cassie Pelvis/RConn2 -- Cassie Right Leg/LConn1
